simulink library "sflib"  (R2025a)
settings: Solver=ode45  StartTime=0.0  StopTime=10.0  RelTol=1e-3  AbsTol=1e-6
settings Model: FPTRunName=Active  ExtModeTrigMode=oneshot  ExtModeArmWhenConnect=off  ExtModeAutoUpdateStatusClock=off  Creator=The MathWorks, Inc.  LastModifiedBy=justi
settings SolverCC: AutoScaleAbsTol=off  AlgebraicLoopSolver=TrustRegion
settings DataIOCC: SaveFormat=Array  SignalLoggingSaveFormat=ModelDataLogs  ReturnWorkspaceOutputs=off  SignalLoggingName=logsOut
settings OptimizationCC: BooleanDataType=off  ReuseModelBlockBuffer=off  ExpressionDepthLimit=2147483647.0  InitFltsAndDblsToZero=on  EfficientMapNaN2IntZero=off  LifeSpan=inf  BufferReusableBoundary=off
settings DebuggingCC: SaveWithParameterizedLinksMsg=none  UnderspecifiedInitializationDetection=Classic  MergeDetectMultiDrivingBlocksExec=none  CheckExecutionContextPreStartOutputMsg=on  SignalResolutionControl=TryResolveAllWithWarning  MultiTaskDSMMsg=warning  MultiTaskCondExecSysMsg=none  IntegerOverflowMsg=none  FcnCallInpInsideContextMsg=warning  UnconnectedInputMsg=warning  UnconnectedOutputMsg=warning  UnconnectedLineMsg=warning  AllowSymbolicDim=off  StateNameClashWarn=warning  SFUnexpectedBacktrackingDiag=warning  SFNoUnconditionalDefaultTransitionDiag=warning  SFExecutionAtInitializationDiag=none  IntegerSaturationMsg=none  ArithmeticOperatorsInVariantConditions=warning
settings HardwareCC: ProdBitPerPointer=32.0  ProdLargestAtomicFloat=None  ProdIntDivRoundTo=Undefined  ProdEndianess=Unspecified  ProdWordSize=32.0  ProdHWDeviceType=32-bit Generic  TargetUnknown=on
settings ModelReferenceCC: UpdateModelReferenceTargets=IfOutOfDate  EnableRefExpFcnMdlSchedulingChecks=on  PropagateSignalLabelsOutOfModel=off
settings SFSimCC: SimUseLocalCustomCode=off  CustomCodeUndefinedFunction=UseInterfaceOnly
settings RTWCC: RTWUseLocalCustomCode=off  GPUComputeCapability=3.5  DLArmComputeVersion=19.05
settings CodeAppCC: StateflowObjectComments=on
settings GRTTargetCC: TargetFcnLib=ansi_tfl_tmw.mat  TargetLangStandard=C89/C90 (ANSI)  CombineOutputUpdateFcns=off  GRTInterface=on
settings ConfigComp: CovMetricSettings=dw  CovSaveCumulativeToWorkspaceVar=on  CovSaveSingleToWorkspaceVar=on  CovExternalEMLEnable=off  CovSFcnEnable=off

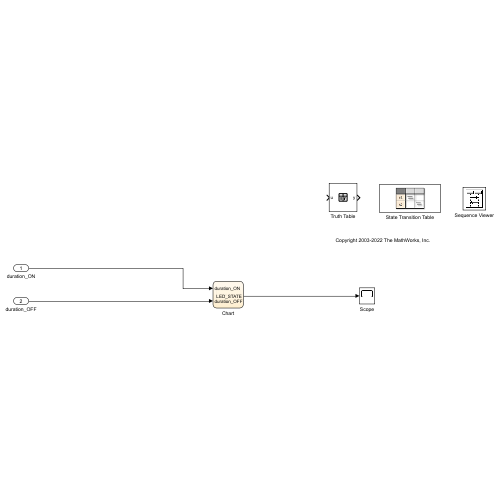
[thumbnail: Simulink's stored preview of the top-level diagram]
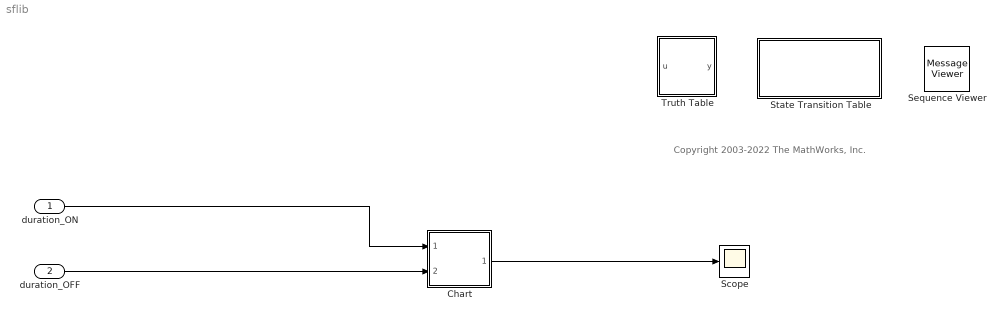
== system sflib ==
  note: Copyright 2003-2022 The MathWorks, Inc.
  duration_ON : Inport  OutMin=1000  OutMax=1000
  duration_OFF : Inport  Port=2  OutMin=1000  OutMax=1000
  Chart : Stateflow chart  BlockKeywords=__PRM__SERIALIZED__DATA__:Stateflow Chart,Stateflow Diagram  TreatAsAtomicUnit=on
  Scope : Scope
      settings: SampleTime=10
  Sequence Viewer : MessageViewer
  State Transition Table : State Transition Table  TreatAsAtomicUnit=on
  Truth Table : Truth Table  TreatAsAtomicUnit=on
  wires:
  Chart/1(LED_STATE) -> Scope/1
  duration_ON/1 -> Chart/1(duration_ON)
  duration_OFF/1 -> Chart/2(duration_OFF)

== matlab function sflib/Truth Table ==
  data: u input; y output
function y = fcn(u)

aVarTruthTableCondition_1 = false;
aVarTruthTableCondition_2 = false;


% Example condition 1

aVarTruthTableCondition_1 = logical(u >= 0);

% Example condition 2

aVarTruthTableCondition_2 = logical(u ^ 2 <= 1);

if (aVarTruthTableCondition_1 && aVarTruthTableCondition_2)
    aFcnTruthTableAction_1();
elseif (~aVarTruthTableCondition_1 && ~aVarTruthTableCondition_2)
    aFcnTruthTableAction_1();
else % Default
    aFcnTruthTableAction_2();
end

function aFcnTruthTableAction_1()

% Example action 1 called from D1 & D2 column in condition table

y = u;

function aFcnTruthTableAction_2()

% Example action 2 called from D3 column in condition table

y = 1 / u;

== stateflow chart sflib/Chart ==
  state ? [group]
    state ? [group]
      state LED_ON
        entry:
        LED_STATE = true
    state LED_OFF
      entry:
      LED_STATE = false
    LED_ON -> LED_OFF : [after(duration_ON, msec)]
    LED_OFF -> LED_ON : [after(duration_OFF, msec)]
  data: duration_ON input; duration_OFF input; LED_STATE output size=1 [0..1]

== stateflow chart sflib/State Transition Table ==
  state state1
  state state2
  (default) -> state1
  state1 -> state2
